simulink model "lab3_100"  (R2020b)
settings: Solver=VariableStepAuto  StartTime=0.0  StopTime=2  RelTol=1e-3
settings Model: Creator=Dexp  LastModifiedBy=takem

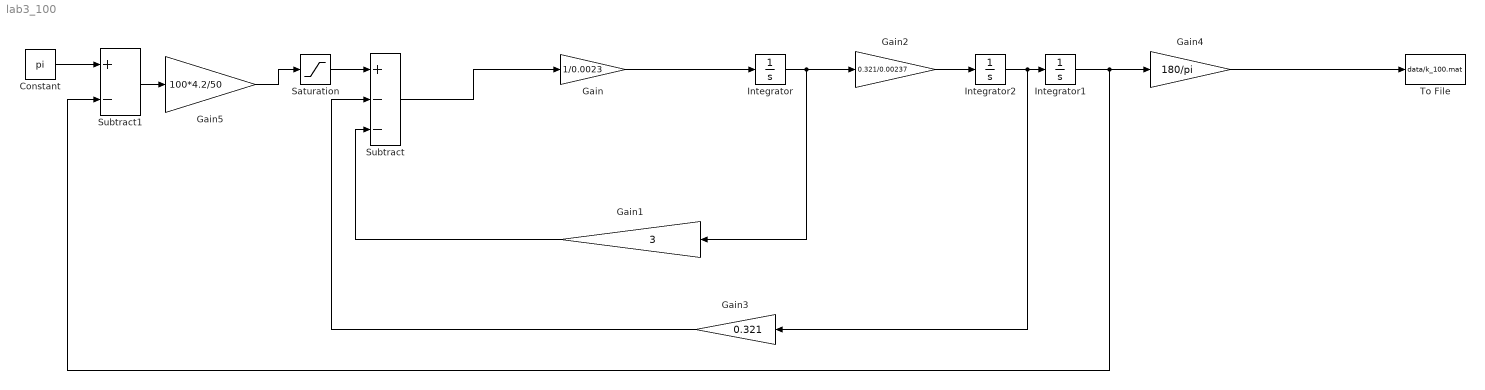
== system lab3_100 ==
  Constant : Constant  Value=pi
  Gain : Gain  Gain=1/0.0023
  Gain1 : Gain  Gain=3
  Gain2 : Gain  Gain=0.321/0.00237
  Gain3 : Gain  Gain=0.321
  Gain4 : Gain  Gain=180/pi
  Gain5 : Gain  Gain=100*4.2/50
  Integrator : Integrator
  Integrator1 : Integrator
  Integrator2 : Integrator
  Saturation : Saturate  UpperLimit=4.3  LowerLimit=-4.3
  Subtract : Sum  Inputs=+--
  Subtract1 : Sum  Inputs=+-
  To File : ToFile  Filename=data/k_100.mat  MatrixName=k_100
  wires:
  Integrator1/1 -> Subtract1/2, Gain4/1
  Subtract/1 -> Gain/1
  Gain/1 -> Integrator/1
  Gain1/1 -> Subtract/3
  Integrator/1 -> Gain2/1, Gain1/1
  Integrator2/1 -> Gain3/1, Integrator1/1
  Gain2/1 -> Integrator2/1
  Gain3/1 -> Subtract/2
  Gain4/1 -> To File/1
  Subtract1/1 -> Gain5/1
  Constant/1 -> Subtract1/1
  Gain5/1 -> Saturation/1
  Saturation/1 -> Subtract/1
